simulink model "Sim31"  (R2019a)
settings: Solver=VariableStepAuto  StartTime=0.0  StopTime=10.0  RelTol=1e-3
settings Model: Creator=fbleo  LastModifiedBy=fbleo

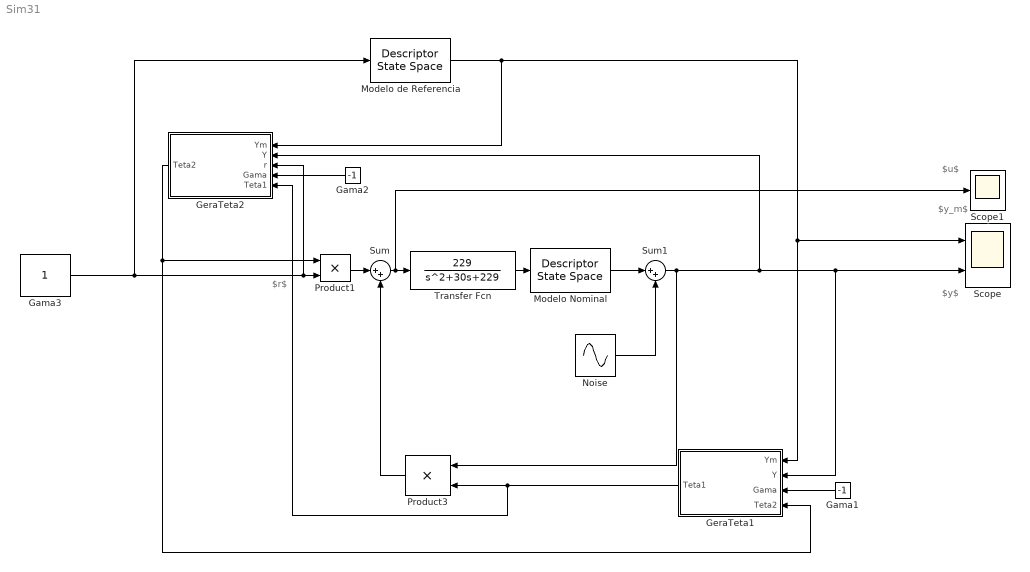
== system Sim31 ==
  note: $r$
  note: $y_m$
  note: $y$
  note: $u$
  Gama1 : Constant  Value=-1
  Gama2 : Constant  Value=-1
  Gama3 : Constant
  GeraTeta1 : Subsystem
  GeraTeta2 : Subsystem
  Modelo Nominal : DescriptorStateSpace  A=-1  B=2  D=0  InitialCondition=0.5
  Modelo de Referencia : DescriptorStateSpace  A=-3  B=3  D=0  InitialCondition=0
  Noise : Sin  Amplitude=0.1  Frequency=16.1  SampleTime=0
  Product1 : Product
  Product3 : Product
  Scope : Scope  NumInputPorts=2
  Scope1 : Scope
  Sum : Sum  Inputs=|++
  Sum1 : Sum  Inputs=|++
  Transfer Fcn : TransferFcn  Numerator=[229]  Denominator=[1 30 229]
  wires:
  Transfer Fcn/1 -> Modelo Nominal/1
  Product1/1 -> Sum/1
  Gama3/1 -> GeraTeta2/3(r), Product1/2, Modelo de Referencia/1
  Product3/1 -> Sum/2
  Gama2/1 -> GeraTeta2/4(Gama)
  GeraTeta2/1(Teta2) -> GeraTeta1/4("Teta2 "), Product1/1
  Modelo de Referencia/1 -> GeraTeta1/1(Ym), Scope/1, GeraTeta2/1(Ym)
  GeraTeta1/1(Teta1) -> GeraTeta2/5("Teta1 "), Product3/2
  Gama1/1 -> GeraTeta1/3(Gama)
  Sum/1 -> Scope1/1, Transfer Fcn/1
  Modelo Nominal/1 -> Sum1/1
  Noise/1 -> Sum1/2
  Sum1/1 -> GeraTeta2/2(Y), GeraTeta1/2(Y), Scope/2, Product3/1

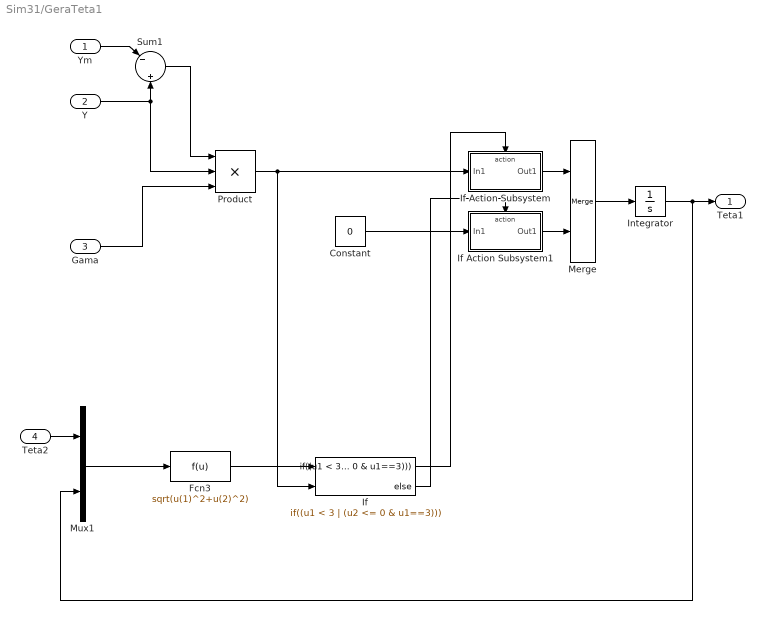
== system Sim31/GeraTeta1 ==
  Ym : Inport
  Y : Inport  Port=2
  Gama : Inport  Port=3
  "Teta2 " : Inport  Port=4
  Constant : Constant  Value=0
  Fcn3 : Fcn  Expr=sqrt(u(1)^2+u(2)^2)
  If : If  NumInputs=2  IfExpression=(u1 < 3 | (u2 <= 0 & u1==3))
  If Action Subsystem : Subsystem  TreatAsAtomicUnit=on
  If Action Subsystem1 : Subsystem  TreatAsAtomicUnit=on
  Integrator : Integrator  InitialCondition=-0.65
  Merge : Merge
  Mux1 : Mux  Inputs=2
  Product : Product  Inputs=3
  Sum1 : Sum  Inputs=|-||+
  Teta1 : Outport
  wires:
  Ym/1 -> Sum1/1
  Sum1/1 -> Product/1
  Y/1 -> Product/2, Sum1/2
  Gama/1 -> Product/3
  Integrator/1 -> Mux1/2, Teta1/1
  Mux1/1 -> Fcn3/1
  "Teta2 "/1 -> Mux1/1
  Fcn3/1 -> If/1
  If/1 -> If Action Subsystem/Action
  Product/1 -> If/2, If Action Subsystem/1(In1)
  If Action Subsystem/1(Out1) -> Merge/1
  Merge/1 -> Integrator/1
  If/2 -> If Action Subsystem1/Action
  If Action Subsystem1/1(Out1) -> Merge/2
  Constant/1 -> If Action Subsystem1/1(In1)

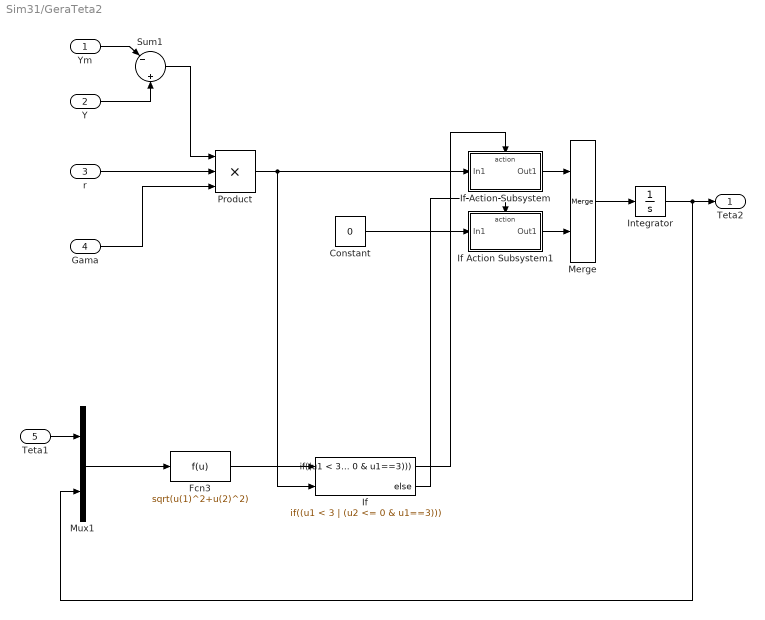
== system Sim31/GeraTeta2 ==
  Ym : Inport
  Y : Inport  Port=2
  r : Inport  Port=3
  Gama : Inport  Port=4
  "Teta1 " : Inport  Port=5
  Constant : Constant  Value=0
  Fcn3 : Fcn  Expr=sqrt(u(1)^2+u(2)^2)
  If : If  NumInputs=2  IfExpression=(u1 < 3 | (u2 <= 0 & u1==3))
  If Action Subsystem : Subsystem  TreatAsAtomicUnit=on
  If Action Subsystem1 : Subsystem  TreatAsAtomicUnit=on
  Integrator : Integrator  InitialCondition=1.14
  Merge : Merge
  Mux1 : Mux  Inputs=2
  Product : Product  Inputs=3
  Sum1 : Sum  Inputs=|-||+
  Teta2 : Outport
  wires:
  Ym/1 -> Sum1/1
  Y/1 -> Sum1/2
  Sum1/1 -> Product/1
  r/1 -> Product/2
  Gama/1 -> Product/3
  Integrator/1 -> Mux1/2, Teta2/1
  Mux1/1 -> Fcn3/1
  "Teta1 "/1 -> Mux1/1
  Fcn3/1 -> If/1
  If/1 -> If Action Subsystem/Action
  Product/1 -> If/2, If Action Subsystem/1(In1)
  If Action Subsystem/1(Out1) -> Merge/1
  Merge/1 -> Integrator/1
  If/2 -> If Action Subsystem1/Action
  If Action Subsystem1/1(Out1) -> Merge/2
  Constant/1 -> If Action Subsystem1/1(In1)

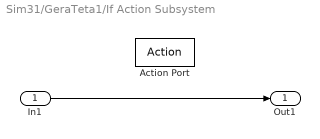
== system Sim31/GeraTeta1/If Action Subsystem ==
  In1 : Inport
  Action Port : ActionPort  ActionPortLabel=if((u1 < 3 | (u2 <= 0 & u1==3)))
  Out1 : Outport
  wires:
  In1/1 -> Out1/1

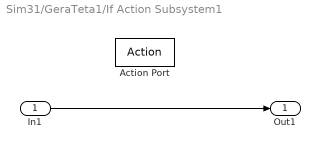
== system Sim31/GeraTeta1/If Action Subsystem1 ==
  In1 : Inport
  Action Port : ActionPort  ActionPortLabel=else
  Out1 : Outport
  wires:
  In1/1 -> Out1/1

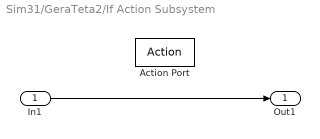
== system Sim31/GeraTeta2/If Action Subsystem ==
  In1 : Inport
  Action Port : ActionPort  ActionPortLabel=if((u1 < 3 | (u2 <= 0 & u1==3)))
  Out1 : Outport
  wires:
  In1/1 -> Out1/1

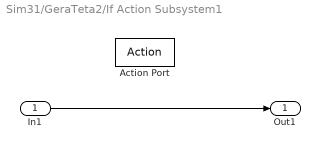
== system Sim31/GeraTeta2/If Action Subsystem1 ==
  In1 : Inport
  Action Port : ActionPort  ActionPortLabel=else
  Out1 : Outport
  wires:
  In1/1 -> Out1/1
